simulink model "ESTbouncing"  (R2017a)
settings: Solver=VariableStepAuto  StartTime=0.0  StopTime=10.0  RelTol=1e-3
settings Model: Creator=xiaodong  LastModifiedBy=xiaodong

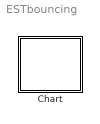
== system ESTbouncing ==
  Chart : Stateflow chart  TreatAsAtomicUnit=on

== stateflow chart ESTbouncing/Chart ==
  state S1
    entry:
    A1 = [1, 0.1; 0 1];
    Bc = [-0.049; -0.9810];
    x =
    during:
  state S2
  (default) -> S1
  data: u1 function_input; u2 function_input; y function_output
  function y = FnM(u1,u2):
    | function y = FnM(u1,u2)
    | y =u1*u2;
